simulink model "factorial"  (R2017b)
settings: Solver=FixedStepDiscrete  StartTime=0.0  StopTime=10.0  RelTol=1e-3
settings Model: Creator=ibrahim  LastModifiedBy=ibrahim
settings OptimizationCC: DefaultParameterBehavior=Inlined  PassReuseOutputArgsAs=Individual arguments
settings DebuggingCC: ParameterTunabilityLossMsg=error
settings SFSimCC: MATLABDynamicMemAlloc=off
settings RTWCC: SystemTargetFile=ert.tlc  GenCodeOnly=on  TemplateMakefile=ert_default_tmf  GenerateReport=on  IncludeHyperlinkInReport=on  LaunchReport=on  GenerateTraceInfo=on  GenerateTraceReport=on  GenerateTraceReportSl=on  GenerateTraceReportSf=on  GenerateTraceReportEml=on  GenerateWebview=on
settings CodeAppCC: ForceParamTrailComments=on  IgnoreCustomStorageClasses=off  OperatorAnnotations=on  SimulinkDataObjDesc=on  SFDataObjDesc=on  InsertBlockDesc=on
settings ERTTargetCC: TargetLangStandard=C99 (ISO)  GenerateSampleERTMain=on  InlinedParameterPlacement=NonHierarchical  ERTCustomFileTemplate=example_file_process.tlc

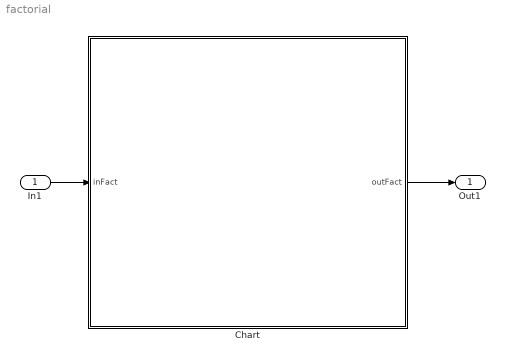
== system factorial ==
  In1 : Inport
  Chart : Stateflow chart  TreatAsAtomicUnit=on
  Out1 : Outport
  wires:
  In1/1 -> Chart/1(inFact)
  Chart/1(outFact) -> Out1/1

== stateflow chart factorial/Chart ==
  (default) -> (junction 6)
  (junction 6) -> (junction 8) : {fact = 1;
      | temp = inFact;}
  (junction 8) -> (junction 16) : /* factorial */
  (junction 16) -> (junction 18)
  (junction 18) -> (junction 17) [order 1] : [temp > 0]
  (junction 17) -> (junction 19) : {fact = fact * temp; temp = temp - 1;}
  (junction 19) -> (junction 18)
  (junction 18) -> (junction 20) [order 2] : {outFact = fact}
  data: inFact input double; outFact output double; fact local double; temp local double
